simulink model "SEDC_controlled_with_rectifier"  (R2023b)
settings: Solver=VariableStepAuto  StartTime=0.0  StopTime=2  FixedStep=1e-3  MaxStep=1e-4  RelTol=1e-3
model workspace (MAT data in the model file):
  Vm = 311.126983722
libraries: spsThyristorLib x4, spsVoltageMeasurementLib x3, spsSeriesRLCBranchLib x2, simulink x2, spsACVoltageSourceLib x1, spsUniversalBridgeLib x1, dspswit3 x1, sps_lib x1
settings Model: NumberOfSteps=800  Creator=gaafa  LastModifiedBy=gaafa

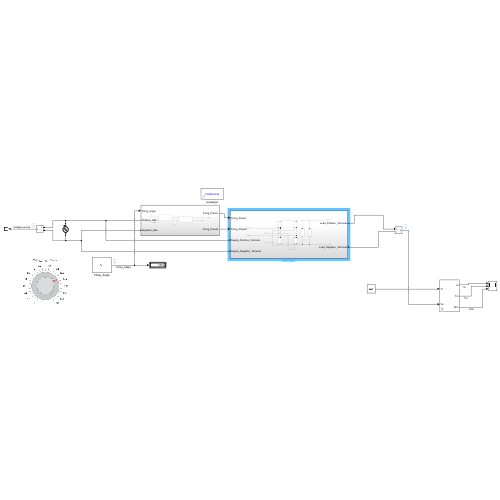
[thumbnail: Simulink's stored preview of the top-level diagram]
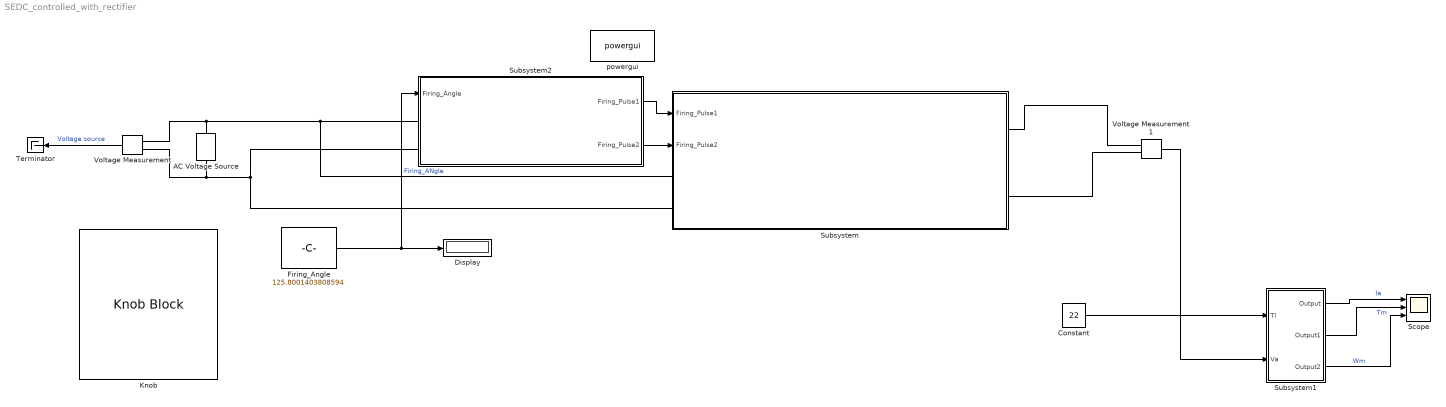
== system SEDC_controlled_with_rectifier ==
  AC Voltage Source : spsACVoltageSourceLib/AC Voltage Source  Amplitude=311.5  Phase=0  Frequency=50  SampleTime=0  Measurements=None  BusType=swing  Pref=10e3  Qref=0  Qmin=-inf  Qmax=+inf
  Constant : Constant  Value=22
  Display : Display
  Firing_Angle : Constant  Value=125.8001403808594
  Knob : KnobBlock  ScaleMax=180
  Scope : Scope  NumInputPorts=3
  Subsystem : Subsystem
  Subsystem1 : Subsystem  mask{La=0.0281, Ra=2.581, J=0.0221, Kf=1.25, B=0.002953}
      mask prompts: La "La (H)"; Ra "Ra (ohm)"; J "J (kg.(m)^2)"; Kf "Kf (V / rad / s)"; B "Bm (N.m.s)"
      mask DialogControl DescGroupVar Prompt: SEDC Motor
      mask DialogControl DescTextVar Prompt: This subsystem is a model for separately excited dc motor
  Subsystem2 : Subsystem
  Terminator : Terminator
  Voltage Measurement : spsVoltageMeasurementLib/Voltage Measurement  PhasorSimulation=off  OutputType=Complex  PSBequivalent=0
  Voltage Measurement1 : spsVoltageMeasurementLib/Voltage Measurement  PhasorSimulation=off  OutputType=Complex  PSBequivalent=0
  powergui : sps_lib/powergui  Priority=1  SimulationMode=Continuous  SampleTime=50e-6  frequency=60  Iterations=50  frequencyindice=0  Pbase=100e6  ErrMax=1e-4  UnitsV=kV  UnitsW=MW  buscounter=0  FunctionMessages=off  echomessages=off  EnableUseOfTLC=off  CurrentSourceSwitches=off  DisableSnubberDevices=off  DisableRonSwitches=off  DisableVfSwitches=off  DisplayEquations=off  AutomaticDiscreteSolvers=off  SolverType=Tustin/Backward Euler (TBE)  Interpol=off  ExternalGateDelay=off  methode=off  Ts=100  x0status=blocks  SPID=on  SwTol=0  HookPort=off  NonlinearTolerance=1e-4  nMaxIteration=100  ContinueOnMaxIteration=off  RestoreLinks=warning  ResistiveCurrentMeasurement=off  Frange=[0:2:500]  Ylog=off  Xlog=on  ShowGrid=off  save=off  variable=ZData  structure=0  ZoomFFT=off  StartTime=0.0  cycles=1  DisplayStyle=1  fundamental=60  FreqAxis=off  MaxFrequency=1000  frequencyindicesteady=1  RmsSteady=1  display=off
  wires:
  Voltage Measurement/1 -> Terminator/1  "Voltage source"
  Firing_Angle/1 -> Subsystem2/1(Firing_Angle), Display/1  "Firing_ANgle"
  Subsystem2/1(Firing_Pulse1) -> Subsystem/1(Firing_Pulse1)
  Subsystem2/2(Firing_Pulse2) -> Subsystem/2(Firing_Pulse2)
  Subsystem1/3(Output2) -> Scope/3  "Wm"
  Constant/1 -> Subsystem1/1(Tl)
  Subsystem1/2(Output1) -> Scope/2  "Tm"
  Subsystem1/1(Output) -> Scope/1  "Ia"
  Voltage Measurement1/1 -> Subsystem1/2(Va)
  connections:
  AC Voltage Source/RConn1 -- Subsystem/LConn1 -- Subsystem2/LConn1 -- Voltage Measurement/LConn1
  AC Voltage Source/LConn1 -- Voltage Measurement/LConn2 -- Subsystem2/LConn2 -- Subsystem/LConn2
  Subsystem/RConn1 -- Voltage Measurement1/LConn1
  Subsystem/RConn2 -- Voltage Measurement1/LConn2

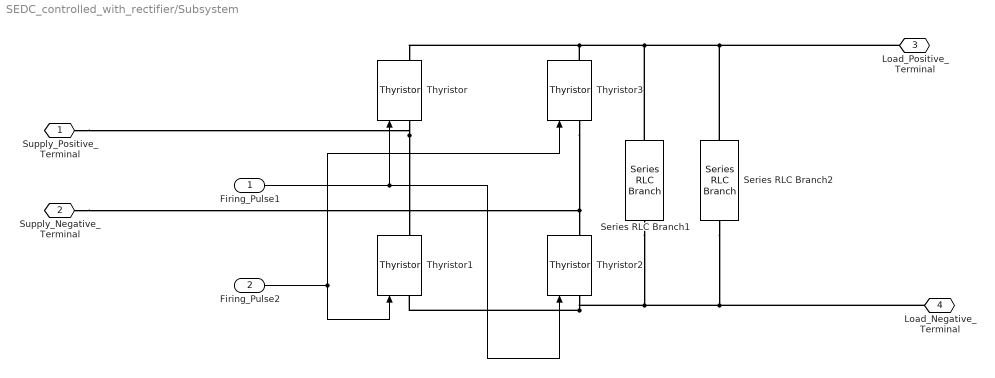
== system SEDC_controlled_with_rectifier/Subsystem ==
  Firing_Pulse1 : Inport
  Firing_Pulse2 : Inport  Port=2
  Series RLC Branch1 : spsSeriesRLCBranchLib/Series RLC Branch  LConnTagsString=__new0  RConnTagsString=__new0  BranchType=R  Resistance=20  Inductance=0.1  SetiL0=off  InitialCurrent=0  Capacitance=.00000005  Setx0=off  InitialVoltage=0  Measurements=None
  Series RLC Branch2 : spsSeriesRLCBranchLib/Series RLC Branch  LConnTagsString=__new0  RConnTagsString=__new0  BranchType=C  Resistance=50  Inductance=6  SetiL0=off  InitialCurrent=0  Capacitance=.5  Setx0=off  InitialVoltage=0  Measurements=None
  Thyristor{,1..3} (4 alike) : spsThyristorLib/Thyristor  Ron=0.001  Lon=0  Vf=0.8  IC=0  Rs=500  Cs=250e-9  Measurements=on
  Supply_Positive_Terminal : PMIOPort  Side=Left
  Supply_Negative_Terminal : PMIOPort  Port=2  Side=Left
  Load_Positive_Terminal : PMIOPort  Port=3  Side=Right
  Load_Negative_Terminal : PMIOPort  Port=4  Side=Right
  wires:
  Firing_Pulse1/1 -> Thyristor2/1, Thyristor/1
  Firing_Pulse2/1 -> Thyristor3/1, Thyristor1/1
  connections:
  Thyristor3/LConn1 -- Thyristor2/RConn1 -- Supply_Negative_Terminal/RConn1
  Thyristor/LConn1 -- Thyristor1/RConn1 -- Supply_Positive_Terminal/RConn1
  Thyristor2/LConn1 -- Series RLC Branch2/RConn1 -- Load_Negative_Terminal/RConn1 -- Series RLC Branch1/RConn1 -- Thyristor1/LConn1
  Thyristor3/RConn1 -- Series RLC Branch2/LConn1 -- Load_Positive_Terminal/RConn1 -- Series RLC Branch1/LConn1 -- Thyristor/RConn1

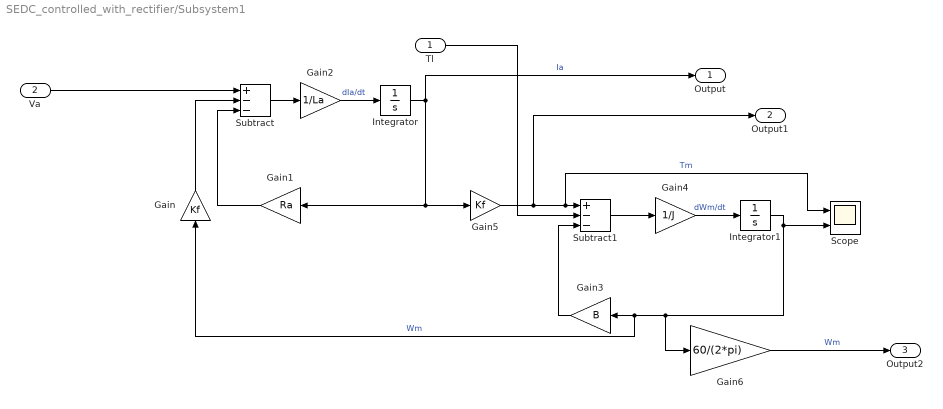
== system SEDC_controlled_with_rectifier/Subsystem1 ==
  Tl : Inport
  Va : Inport  Port=2
  Gain : Gain  Gain=Kf
  Gain1 : Gain  Gain=Ra
  Gain2 : Gain  Gain=1/La
  Gain3 : Gain  Gain=B
  Gain4 : Gain  Gain=1/J
  Gain5 : Gain  Gain=Kf
  Gain6 : Gain  Gain=60/(2*pi)
  Integrator : Integrator
  Integrator1 : Integrator
  Scope : Scope  NumInputPorts=2
  Subtract : Sum  Inputs=+--
  Subtract1 : Sum  Inputs=+--
  Output : Outport
  Output1 : Outport  Port=2
  Output2 : Outport  Port=3
  wires:
  Integrator/1 -> Output/1, Gain5/1, Gain1/1  "Ia"
  Gain5/1 -> Output1/1, Scope/1, Subtract1/1  "Tm"
  Integrator1/1 -> Scope/2, Gain6/1, Gain/1, Gain3/1  "Wm"
  Gain2/1 -> Integrator/1  "dIa/dt"
  Tl/1 -> Subtract1/2
  Gain1/1 -> Subtract/3
  Subtract/1 -> Gain2/1
  Gain/1 -> Subtract/2
  Gain3/1 -> Subtract1/3
  Gain4/1 -> Integrator1/1  "dWm/dt"
  Subtract1/1 -> Gain4/1
  Va/1 -> Subtract/1
  Gain6/1 -> Output2/1  "Wm"

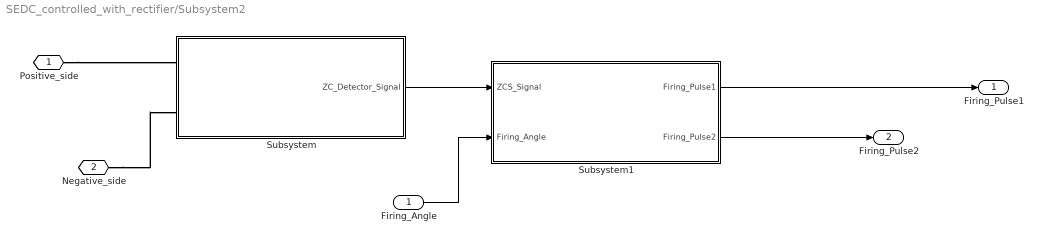
== system SEDC_controlled_with_rectifier/Subsystem2 ==
  Firing_Angle : Inport
  Subsystem : Subsystem
  Subsystem1 : Subsystem
  Positive_side : PMIOPort  Side=Left
  Negative_side : PMIOPort  Port=2  Side=Left
  Firing_Pulse1 : Outport
  Firing_Pulse2 : Outport  Port=2
  wires:
  Subsystem/1(ZC_Detector_Signal) -> Subsystem1/1(ZCS_Signal)
  Subsystem1/1(Firing_Pulse1) -> Firing_Pulse1/1
  Firing_Angle/1 -> Subsystem1/2(Firing_Angle)
  Subsystem1/2(Firing_Pulse2) -> Firing_Pulse2/1
  connections:
  Positive_side/RConn1 -- Subsystem/LConn1
  Negative_side/RConn1 -- Subsystem/LConn2

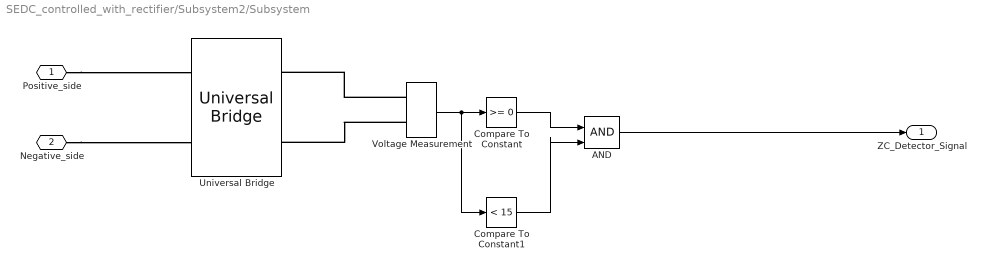
== system SEDC_controlled_with_rectifier/Subsystem2/Subsystem ==
  AND : Logic  IconShape=distinctive  AllPortsSameDT=off  OutDataTypeStr=boolean
  Compare To Constant : simulink/Logic and Bit Operations/Compare To Constant  relop=>=  const=0  OutDataTypeStr=boolean
  Compare To Constant1 : simulink/Logic and Bit Operations/Compare To Constant  relop=<  const=15  OutDataTypeStr=boolean
  Universal Bridge : spsUniversalBridgeLib/Universal Bridge  Arms=2  SnubberResistance=1e5  SnubberCapacitance=inf  Device=Diodes  Ron=1e-3  Lon=0  ForwardVoltages="[  0  0  ]"  ForwardVoltage=0  GTOparameters=[ 10e-6 , 20e-6 ]  IGBTparameters=[ 1e-6 , 2e-6 ]  Measurements=None  Measurements_2=None  converterType=Rectifier
  Voltage Measurement : spsVoltageMeasurementLib/Voltage Measurement  PhasorSimulation=off  OutputType=Complex  PSBequivalent=0
  Positive_side : PMIOPort  Side=Left
  Negative_side : PMIOPort  Port=2  Side=Left
  ZC_Detector_Signal : Outport
  wires:
  Compare To Constant/1 -> AND/1
  AND/1 -> ZC_Detector_Signal/1
  Voltage Measurement/1 -> Compare To Constant1/1, Compare To Constant/1
  Compare To Constant1/1 -> AND/2
  connections:
  Positive_side/RConn1 -- Universal Bridge/LConn1
  Negative_side/RConn1 -- Universal Bridge/LConn2
  Voltage Measurement/LConn1 -- Universal Bridge/RConn1
  Voltage Measurement/LConn2 -- Universal Bridge/RConn2

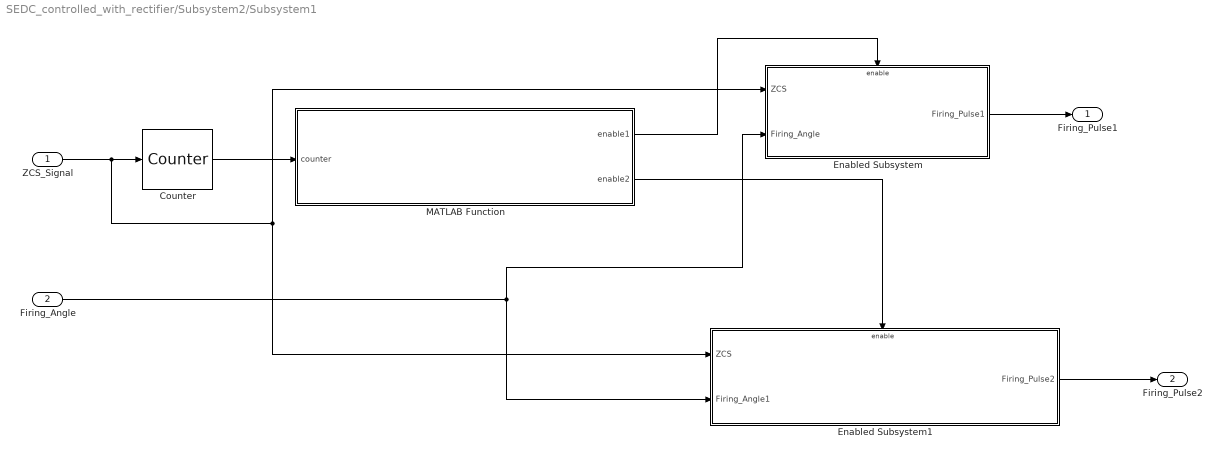
== system SEDC_controlled_with_rectifier/Subsystem2/Subsystem1 ==
  ZCS_Signal : Inport
  Firing_Angle : Inport  Port=2
  Counter : dspswit3/Counter  Direction=Up  CountEvent=Rising edge  CounterSize=User defined  MaxCount=255  InitialCount=0  Output=Count  HitValue=32  ResetInput=off  SamplesPerFrame=1  Ts=1  CntDtype=double  HitDtype=Logical
  Enabled Subsystem : Subsystem  TreatAsAtomicUnit=on
  Enabled Subsystem1 : Subsystem  TreatAsAtomicUnit=on
  MATLAB Function : MATLAB Function  TreatAsAtomicUnit=on
  Firing_Pulse1 : Outport
  Firing_Pulse2 : Outport  Port=2
  wires:
  ZCS_Signal/1 -> Enabled Subsystem/1(ZCS), Enabled Subsystem1/1(ZCS), Counter/1
  Counter/1 -> MATLAB Function/1(counter)
  MATLAB Function/1(enable1) -> Enabled Subsystem/Enable
  MATLAB Function/2(enable2) -> Enabled Subsystem1/Enable
  Firing_Angle/1 -> Enabled Subsystem/2(Firing_Angle), Enabled Subsystem1/2(Firing_Angle1)
  Enabled Subsystem/1(Firing_Pulse1) -> Firing_Pulse1/1
  Enabled Subsystem1/1(Firing_Pulse2) -> Firing_Pulse2/1

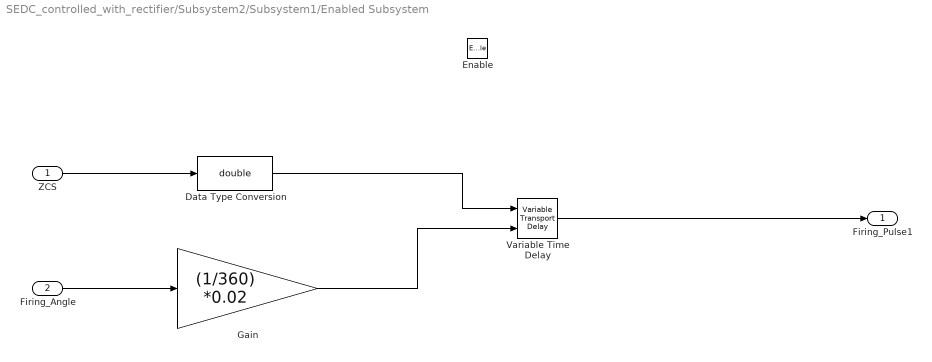
== system SEDC_controlled_with_rectifier/Subsystem2/Subsystem1/Enabled Subsystem ==
  ZCS : Inport
  Firing_Angle : Inport  Port=2
  Enable : EnablePort
  Data Type Conversion : DataTypeConversion  OutDataTypeStr=double  SaturateOnIntegerOverflow=off  RndMeth=Floor
  Gain : Gain  Gain=(1/360) *0.02
  Variable Time Delay : VariableTransportDelay  MaximumDelay=10
  Firing_Pulse1 : Outport
  wires:
  ZCS/1 -> Data Type Conversion/1
  Data Type Conversion/1 -> Variable Time Delay/1
  Firing_Angle/1 -> Gain/1
  Gain/1 -> Variable Time Delay/2
  Variable Time Delay/1 -> Firing_Pulse1/1

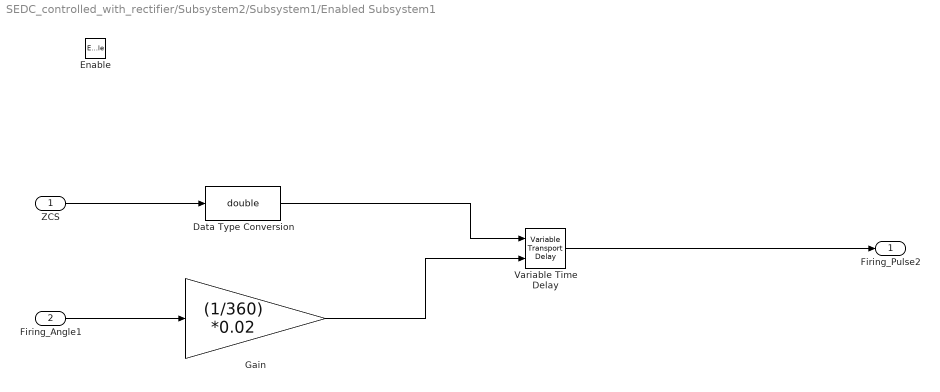
== system SEDC_controlled_with_rectifier/Subsystem2/Subsystem1/Enabled Subsystem1 ==
  ZCS : Inport
  Firing_Angle1 : Inport  Port=2
  Enable : EnablePort
  Data Type Conversion : DataTypeConversion  OutDataTypeStr=double  SaturateOnIntegerOverflow=off  RndMeth=Floor
  Gain : Gain  Gain=(1/360) *0.02
  Variable Time Delay : VariableTransportDelay  MaximumDelay=10
  Firing_Pulse2 : Outport
  wires:
  Gain/1 -> Variable Time Delay/2
  Variable Time Delay/1 -> Firing_Pulse2/1
  Firing_Angle1/1 -> Gain/1
  ZCS/1 -> Data Type Conversion/1
  Data Type Conversion/1 -> Variable Time Delay/1

== matlab function SEDC_controlled_with_rectifier/Subsystem2/Subsystem1/MATLAB Function ==
  data: counter input; enable1 output; enable2 output
function [enable1 , enable2] = Pulse_Generator(counter)
enable1 = 0;
enable2 = 0;
if (mod(counter , 2 ) == 0)
    enable1 = 1;
    enable2 = 0;
end


if (mod(counter , 2 ) == 1)
    enable1 = 0;
    enable2 = 1;
end

end
